simulink model "INTER_IIT_order_4_DSM"  (R2024a)
settings: Solver=FixedStepDiscrete  StartTime=0.0  StopTime=4.608  RelTol=1e-3
undefined symbols (not defined in the file): DiscIntNeverNeededParam
settings Model: Creator=Siddhant  LastModifiedBy=Siddhant

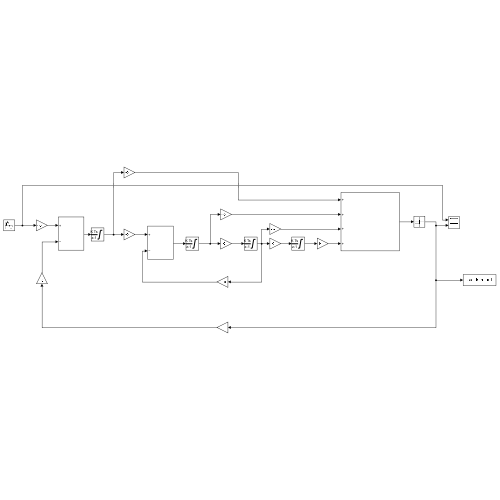
[thumbnail: Simulink's stored preview of the top-level diagram]
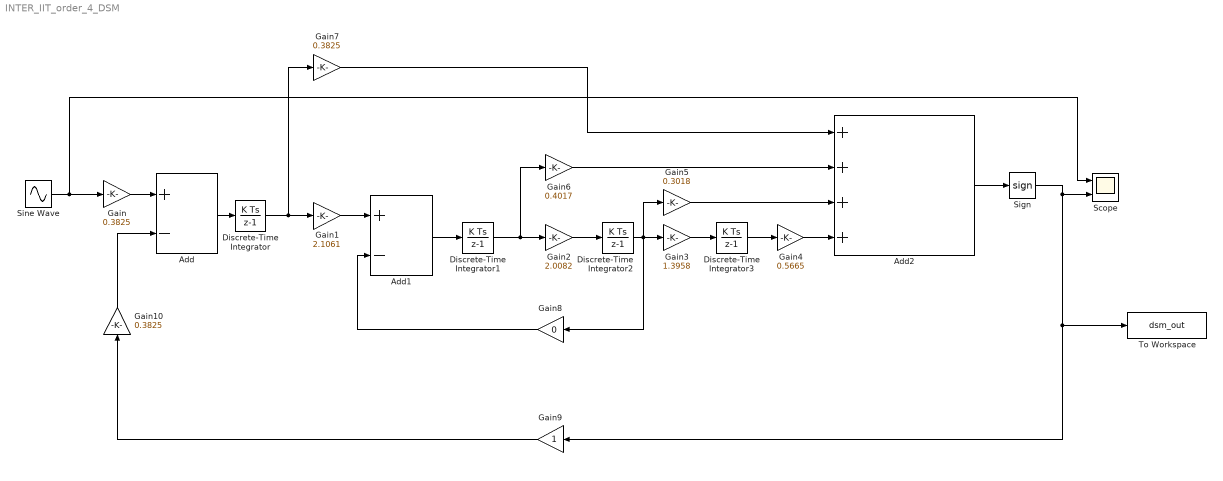
== system INTER_IIT_order_4_DSM ==
  Add : Sum  Inputs=+-
  Add1 : Sum  Inputs=+-
  Add2 : Sum  Inputs=++++
  Discrete-Time Integrator{,1..3} (4 alike) : DiscreteIntegrator  SampleTime=1/8.192e6  LimitOutput=on  UpperSaturationLimit=1.8  LowerSaturationLimit=-1.8  ICPrevOutput=DiscIntNeverNeededParam  ICPrevScaledInput=DiscIntNeverNeededParam
  Gain : Gain  Gain=0.3825
  Gain1 : Gain  Gain=2.1061
  Gain10 : Gain  Gain=0.3825
  Gain2 : Gain  Gain=2.0082
  Gain3 : Gain  Gain=1.3958
  Gain4 : Gain  Gain=0.5665
  Gain5 : Gain  Gain=0.3018
  Gain6 : Gain  Gain=0.4017
  Gain7 : Gain  Gain=0.3825
  Gain8 : Gain  Gain=0
  Gain9 : Gain
  Scope : Scope  NumInputPorts=2
  Sign : Signum
  Sine Wave : Sin  Amplitude=0.9  Frequency=4712.39  Samples=163660  SampleTime=1/8.192e6
  To Workspace : ToWorkspace  VariableName=dsm_out  SampleTime=-1
  wires:
  Gain/1 -> Add/1
  Add/1 -> Discrete-Time Integrator/1
  Discrete-Time Integrator/1 -> Gain7/1, Gain1/1
  Gain1/1 -> Add1/1
  Add1/1 -> Discrete-Time Integrator1/1
  Discrete-Time Integrator1/1 -> Gain6/1, Gain2/1
  Gain2/1 -> Discrete-Time Integrator2/1
  Discrete-Time Integrator2/1 -> Gain8/1, Gain5/1, Gain3/1
  Gain3/1 -> Discrete-Time Integrator3/1
  Discrete-Time Integrator3/1 -> Gain4/1
  Gain4/1 -> Add2/4
  Gain5/1 -> Add2/3
  Gain6/1 -> Add2/2
  Gain7/1 -> Add2/1
  Add2/1 -> Sign/1
  Gain8/1 -> Add1/2
  Gain10/1 -> Add/2
  Gain9/1 -> Gain10/1
  Sign/1 -> Gain9/1, To Workspace/1, Scope/2
  Sine Wave/1 -> Scope/1, Gain/1
